simulink model "SiEngineCore"  (R2017b)
settings: Solver=VariableStepAuto  StartTime=0.0  StopTime=inf  RelTol=1e-3  EnableMultiTasking=on
model workspace (MAT data in the model file):
  AFRStoich = 14.6
  AirFilterArea = 0.000962112750162
  AirIntakeVol = 0.0137
  C_eng = 40000
  CompEff = [0.2 0.2 0.2 0.2 0.2 0.2 0.2 0.2 0.2 0.2 0.2 0.2 ... (5000 elements, 50x100)]
  CompMassFlwRate = [4.4091251837e-05 0.00441685548409 0.00879200250921 0.0131688186568 0.0175465480563 0.0219243905675 0.0263014996182 0.0306769799437 0.0350498852261 0.0394192156283 0.0437839152204 0.0481428692931 ... (5000 elements, 50x100)]
  CompPrsRatioBreakPoints = [1 1.02808080808 1.05616161616 1.08424242424 1.11232323232 1.1404040404 1.16848484848 1.19656565657 1.22464646465 1.25272727273 1.28080808081 1.30888888889 ... (100 elements, 1x100)]
  CompRefPrs = 101325
  CompRefTemp = 300
  CompSpdBreakPoints = [5 500.713942607 996.427885215 1492.14182782 1987.85577043 2483.56971304 2979.28365564 3474.99759825 3970.71154086 4466.42548347 4962.13942607 5457.85336868 ... (50 elements, 1x50)]
  CoolantTemp = 310
  Cps = 2
  ExhSysArea = 0.00138544236023
  ExhSysVol = 0.0044
  IcEffectiveness = 0.7
  InjSlp = 6.45161290323
  LHV = 47300000
  NCyl = 4
  Pstd = 101325
  Rair = 287
  Rexh = 297
  T_cool_start = 355
  T_coolnt_init = 355
  T_coolnt_max = 375
  ThrAngToC = [0  0.001; 90  0.735]
  ThrDiam = 50
  Tstd = 293.15
  TurbEff = [0.1 0.1 0.1 0.1 0.1 0.1 0.1 0.1 0.1 0.1 0.1 0.1 ... (3600 elements, 60x60)]
  TurbMassFlwRate = [0 0 0 0 0 0 0 0 0 0 0 0 ... (3600 elements, 60x60)]
  TurbPrsRatioBreakPoints = [1 1.0066198 1.0187236 1.0343974 1.0529583 1.0740113 1.0972904 1.1226 1.1497884 1.178734 1.2093357 1.2415084 ... (60 elements, 1x60)]
  TurbRefPres = 101325
  TurbRefTemp = 300
  TurbSpdBreakPoints = [0 236.716179913 473.432359826 710.148557878 946.864755929 1183.5809177 1420.29711576 1657.01327753 1893.72933048 2130.44574618 2367.16179913 2603.87821484 ... (60 elements, 60x1)]
  TurboInertia = 1.55e-05
  Vd = 0.0015
  Vexh = 0.0016
  Vint = 0.00286
  VolCompOut = 0.0026
  WgArea = 0.000314159265359
  cp_air = 1005
  cp_exh = 1005
  f_co = [6.86026635502e-05 6.86026635502e-05 0.000137130178455 0.000177313004818 0.000153545722458 0.000286109103754 0.00065603982686 0.00012726330728 0.000129286672759 0.000129286672759 0.000129286672759 0.000129286672759 ... (240 elements, 16x15)]
  f_co2 = [0.190124640361 0.190124640361 0.197310430134 0.198841052192 0.19976911847 0.200569885042 0.199664821109 0.20034918367 0.20035007673 0.20035007673 0.20035007673 0.20035007673 ... (240 elements, 16x15)]
  f_del_sa_bpt = [0 0.75 1.5 2.25 3 3.75 4.5 5.25 6 6.75 7.5 8.25 ... (65 elements, 1x65)]
  f_exhfrac_n_bpt = [750 1053.57142857 1357.14285714 1660.71428571 1964.28571429 2267.85714286 2571.42857143 2875 3178.57142857 3482.14285714 3785.71428571 4089.28571429 ... (15 elements, 1x15)]
  f_exhfrac_trq_bpt = [0 15 26.4285714286 37.8571428571 49.2857142857 60.7142857143 72.1428571429 83.5714285714 95 106.428571429 117.857142857 129.285714286 ... (16 elements, 1x16)]
  f_fric_temp_bpt = [274 276 278 280 282 284 286 288 290 292 294 296 ... (54 elements, 1x54)]
  f_fric_temp_mod = [3.96 3.22 2.56 2.26 2.11 2 1.9 1.83 1.76 1.7 1.65 1.6 ... (54 elements, 1x54)]
  f_hc = [0.00443209119576 0.00443209119576 0.00220684816441 0.00166684424867 0.00138421884093 0.0010658858934 0.00112857643245 0.00117703080332 0.00117597584116 0.00117597584116 0.00117597584116 0.00117597584116 ... (240 elements, 16x15)]
  f_m_lam = [0.94128 0.95565 0.97001 0.98437 0.99008 1.0004 0.97527 0.9549 0.92612 0.89735 0]
  f_m_lam_bpt = [0.65 0.7 0.75 0.8 0.85 0.9 0.95 1 1.05 1.1 2]
  f_m_sa = [1.0019 0.9988 0.9953 0.99173 0.98811 0.98441 0.98065 0.97682 0.97293 0.96897 0.96493 0.96083 ... (65 elements, 1x65)]
  f_mdot_air = [0 0 0 0 0 0 0 0 0 0 0 0 ... (400 elements, 20x20)]
  f_mdot_air_corr = [1.02156051768 1.00597426471 0.989411677851 1.0033499089 0.984591437857 0.988509040623 1.0326198627 1.02765527362 1.0134784519 0.998280021213 0.981755128787 0.967218261288 ... (400 elements, 20x20)]
  f_mdot_air_corr_ld_bpt = [0.223381333333 0.285105122807 0.346828912281 0.408552701754 0.470276491228 0.532000280702 0.593724070175 0.655447859649 0.717171649123 0.778895438596 0.84061922807 0.902343017544 ... (20 elements, 1x20)]
  f_mdot_air_ecp_bpt = [0 2.6316 5.2632 7.8947 10.5263 13.1579 15.7895 18.4211 21.0526 23.6842 26.3158 28.9474 ... (20 elements, 1x20)]
  f_mdot_air_n_bpt = [750 973.6842 1197.3684 1421.0526 1644.7368 1868.4211 2092.1053 2315.7895 2539.4737 2763.1579 2986.8421 3210.5263 ... (20 elements, 1x20)]
  f_mdot_trpd_bpt = [0 5.7895 11.5789 17.3684 23.1579 28.9474 34.7368 40.5263 46.3158 52.1053 57.8947 63.6842 ... (20 elements, 1x20)]
  f_nox = [4.08881357131e-05 4.08881357131e-05 0.00012346903723 0.000189339284589 0.00026637780763 0.000608287545555 0.00102018770254 0.00131576653087 0.00131610412986 0.00131610412986 0.00131610412986 0.00131610412986 ... (240 elements, 16x15)]
  f_nv = [0.64175366561 0.641419295169 0.640125365558 0.638690556197 0.644169906538 0.669178791311 0.731659452876 0.750078238889 0.750078238889 0.750078238889 0.750078238889 0.750078238889 ... (225 elements, 15x15)]
  f_nv_n_bpt = [750 1053.57142857 1357.14285714 1660.71428571 1964.28571429 2267.85714286 2571.42857143 2875 3178.57142857 3482.14285714 3785.71428571 4089.28571429 ... (15 elements, 1x15)]
  f_nv_prs_bpt = [31 40.6428571429 50.2857142857 59.9285714286 69.5714285714 79.2142857143 88.8571428571 98.5 108.142857143 117.785714286 127.428571429 137.071428571 ... (15 elements, 1x15)]
  f_sa_opt = [35.3085 35.3085 21.0105 10.3714 8.5076 7.1426 7.5656 -5.7766 -16.7061 -16.8345 -19.3546 -20.6085 ... (256 elements, 16x16)]
  f_t_exh = [739.936218766 750.584766028 772.770773797 791.235245621 803.106549716 885.862998064 920.498479307 920.498479307 920.498479307 920.498479307 920.498479307 920.498479307 ... (225 elements, 15x15)]
  f_t_exh_l_bpt = [0.2 0.275 0.35 0.425 0.5 0.575 0.65 0.725 0.8 0.875 0.95 1.025 ... (15 elements, 1x15)]
  f_t_exh_n_bpt = [750 1053.57142857 1357.14285714 1660.71428571 1964.28571429 2267.85714286 2571.42857143 2875 3178.57142857 3482.14285714 3785.71428571 4089.28571429 ... (15 elements, 1x15)]
  f_tm_corr = [0.839360054391 0.833393271885 0.82629554201 0.818442814437 0.811524387436 0.809164184856 0.814606352881 0.826887956871 0.842304598924 0.856886829014 0.869487025783 0.880530414174 ... (400 elements, 20x20)]
  f_tm_corr_n_bpt = [750 973.6842 1197.3684 1421.0526 1644.7368 1868.4211 2092.1053 2315.7895 2539.4737 2763.1579 2986.8421 3210.5263 ... (20 elements, 1x20)]
  f_tm_corr_nd_bpt = [0.3 0.38947 0.47895 0.56842 0.65789 0.74737 0.83684 0.92632 1.0158 1.1053 1.1947 1.2842 ... (20 elements, 1x20)]
  f_tq_fric = [0 0 0 0 0 0 0 0 0 0 0 0 ... (256 elements, 16x16)]
  f_tq_inr = [25.8508 25.8508 25.8508 25.8508 25.8508 25.8508 25.8508 25.8508 25.8508 25.8508 25.8508 25.8508 ... (256 elements, 16x16)]
  f_tq_inr_l_bpt = [0.1 0.2 0.28571 0.37143 0.45714 0.54286 0.62857 0.71429 0.8 0.88571 0.97143 1.0571 ... (16 elements, 1x16)]
  f_tq_inr_n_bpt = [0 750 1053.5714 1357.1429 1660.7143 1964.2857 2267.8571 2571.4286 2875 3178.5714 3482.1429 3785.7143 ... (16 elements, 1x16)]
  f_tq_nl = [15.0012133443 26.4298333923 37.8556656512 49.2846782956 60.7113978793 72.3451969202 77.459652163 78.5324534074 78.5324534074 78.5324534074 78.5324534074 78.5324534074 ... (225 elements, 15x15)]
  f_tq_nl_l_bpt = [0.2 0.275 0.35 0.425 0.5 0.575 0.65 0.725 0.8 0.875 0.95 1.025 ... (15 elements, 1x15)]
  f_tq_nl_n_bpt = [750 1053.57142857 1357.14285714 1660.71428571 1964.28571429 2267.85714286 2571.42857143 2875 3178.57142857 3482.14285714 3785.71428571 4089.28571429 ... (15 elements, 1x15)]
  f_tq_pump = [0 0 0 0 0 0 0 0 0 0 0 0 ... (256 elements, 16x16)]
  f_vivc = [0.37716 0.38164 0.38611 0.39033 0.39428 0.39795 0.40132 0.40441 0.40719 0.40967 0.41184 0.41372 ... (20 elements, 1x20)]
  f_vivc_icp_bpt = [0 2.6316 5.2632 7.8947 10.5263 13.1579 15.7895 18.4211 21.0526 23.6842 26.3158 28.9474 ... (20 elements, 1x20)]
  tau_cool = 3000
libraries: autolibfundflw x11, autolibboost x3, simulink x1, autolibcoreeng x1
(part 2 of 2)

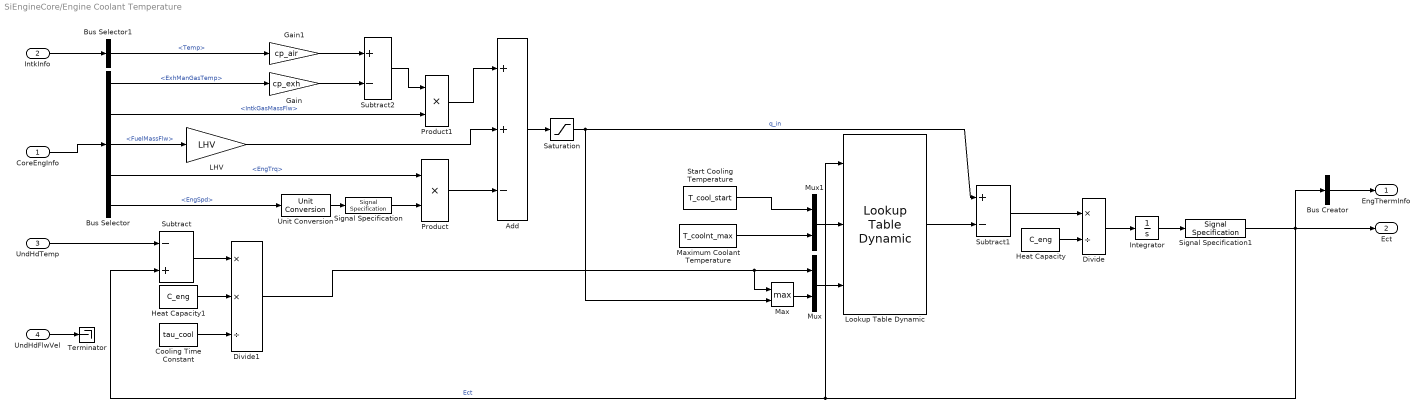
== system SiEngineCore/Engine Coolant Temperature ==
  CoreEngInfo : Inport
  IntkInfo : Inport  Port=2
  UndHdTemp : Inport  Port=3
  UndHdFlwVel : Inport  Port=4
  Add : Sum  Inputs=++-
  Bus Creator : BusCreator  Inputs=1
  Bus Selector : BusSelector  OutputSignals=ExhManGasTemp,IntkGasMassFlw,FuelMassFlw,EngTrq,EngSpd
  Bus Selector1 : BusSelector  OutputSignals=Vol.Temp
  Cooling Time Constant : Constant  Value=tau_cool
  Divide : Product  Inputs=*/
  Divide1 : Product  Inputs=**/
  Gain : Gain  Gain=cp_exh
  Gain1 : Gain  Gain=cp_air
  Heat Capacity : Constant  Value=C_eng
  Heat Capacity1 : Constant  Value=C_eng
  Integrator : Integrator  InitialCondition=T_coolnt_init  LimitOutput=on  UpperSaturationLimit=T_coolnt_max  LowerSaturationLimit=0  ZeroCross=off
  LHV : Gain  Gain=LHV
  Lookup Table Dynamic : simulink/Lookup Tables/Lookup Table Dynamic  LookUpMeth=Interpolation-Use End Values  OutDataType=fixdt('double')  OutScaling=[]  OutputDataTypeScalingMode=Specify via dialog  OutDataTypeStr=double  DoSatur=off
      settings: SourceProductName=Simulink
  Max : MinMax  Function=max  Inputs=2  ZeroCross=off
  Maximum Coolant Temperature : Constant  Value=T_coolnt_max
  Mux : Mux  Inputs=2
  Mux1 : Mux  Inputs=2
  Product : Product
  Product1 : Product
  Saturation : Saturate  UpperLimit=Inf  LowerLimit=0
  Signal Specification : SignalSpecification  Unit=rad/s
  Signal Specification1 : SignalSpecification  Unit=K
  Start Cooling Temperature : Constant  Value=T_cool_start
  Subtract : Sum  Inputs=-+
  Subtract1 : Sum  Inputs=+-
  Subtract2 : Sum  Inputs=+-
  Terminator : Terminator
  Unit Conversion : UnitConversion
  EngThermInfo : Outport  Unit=K
  Ect : Outport  Port=2  Unit=K
  wires:
  UndHdTemp/1 -> Subtract/1
  Heat Capacity/1 -> Divide/2
  Unit Conversion/1 -> Signal Specification/1
  Maximum Coolant Temperature/1 -> Mux1/2
  Signal Specification1/1 -> Subtract/2, Lookup Table Dynamic/1, Bus Creator/1, Ect/1  "Ect"
  UndHdFlwVel/1 -> Terminator/1
  Gain/1 -> Subtract2/2
  Bus Selector/4 -> Product/1  "<EngTrq>"
  Mux1/1 -> Lookup Table Dynamic/2
  Divide1/1 -> Max/1, Mux/1
  Heat Capacity1/1 -> Divide1/2
  Mux/1 -> Lookup Table Dynamic/3
  Start Cooling Temperature/1 -> Mux1/1
  Subtract/1 -> Divide1/1
  Saturation/1 -> Max/2, Subtract1/1  "q_in"
  Signal Specification/1 -> Product/2
  LHV/1 -> Add/2
  Product/1 -> Add/3
  Bus Selector/5 -> Unit Conversion/1  "<EngSpd>"
  Cooling Time Constant/1 -> Divide1/3
  CoreEngInfo/1 -> Bus Selector/1
  Bus Selector/3 -> LHV/1  "<FuelMassFlw>"
  Bus Selector/1 -> Gain/1  "<ExhManGasTemp>"
  Gain1/1 -> Subtract2/1
  Bus Selector1/1 -> Gain1/1  "<Temp>"
  Divide/1 -> Integrator/1
  Subtract1/1 -> Divide/1
  Lookup Table Dynamic/1 -> Subtract1/2
  Max/1 -> Mux/2
  Bus Creator/1 -> EngThermInfo/1
  IntkInfo/1 -> Bus Selector1/1
  Integrator/1 -> Signal Specification1/1
  Subtract2/1 -> Product1/1
  Bus Selector/2 -> Product1/2  "<IntkGasMassFlw>"
  Product1/1 -> Add/1
  Add/1 -> Saturation/1

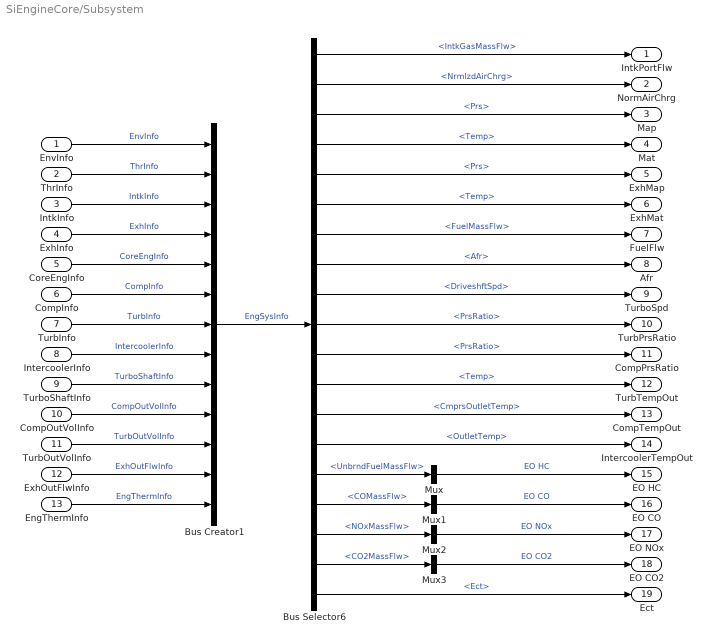
== system SiEngineCore/Subsystem ==
  EnvInfo : Inport
  ThrInfo : Inport  Port=2
  IntkInfo : Inport  Port=3
  ExhInfo : Inport  Port=4
  CoreEngInfo : Inport  Port=5
  CompInfo : Inport  Port=6
  TurbInfo : Inport  Port=7
  IntercoolerInfo : Inport  Port=8
  TurboShaftInfo : Inport  Port=9
  CompOutVolInfo : Inport  Port=10
  TurbOutVolInfo : Inport  Port=11
  ExhOutFlwInfo : Inport  Port=12
  EngThermInfo : Inport  Port=13
  Bus Creator1 : BusCreator  Inputs=13
  Bus Selector6 : BusSelector  OutputSignals=CoreEngInfo.IntkGasMassFlw,CoreEngInfo.NrmlzdAirChrg,IntkInfo.Vol.Prs,IntkInfo.Vol.Temp,ExhInfo.Vol.Prs,ExhInfo.Vol.Temp,CoreEngInfo.FuelMassFlw,CoreEngInfo.Afr,TurboShaftInfo.DriveshftSpd,TurbInfo.PrsRatio,CompInfo.PrsRatio,TurbOutVolInfo.Vol.Temp,CompInfo.CmprsOutletTemp,IntercoolerInfo.OutletTemp,ExhOutFlwInfo.Flw.Species.UnbrndFuelMassFlw,ExhOutFlwInfo.Flw.Species.COMassFlw,ExhOutFlwInfo.Flw.Species.NOxMassFlw,ExhOutFlwInfo.Flw.Species.CO2MassFlw,EngThermInfo.Ect
  Mux{,1..3} (4 alike) : Mux  Inputs=1
  IntkPortFlw : Outport
  NormAirChrg : Outport  Port=2  Unit=1
  Map : Outport  Port=3
  Mat : Outport  Port=4
  ExhMap : Outport  Port=5
  ExhMat : Outport  Port=6
  FuelFlw : Outport  Port=7
  Afr : Outport  Port=8  Unit=1
  TurboSpd : Outport  Port=9
  TurbPrsRatio : Outport  Port=10
  CompPrsRatio : Outport  Port=11
  TurbTempOut : Outport  Port=12
  CompTempOut : Outport  Port=13
  IntercoolerTempOut : Outport  Port=14
  EO HC : Outport  Port=15
  EO CO : Outport  Port=16
  EO NOx : Outport  Port=17
  EO CO2 : Outport  Port=18
  Ect : Outport  Port=19
  wires:
  CompInfo/1 -> Bus Creator1/6  "CompInfo"
  IntkInfo/1 -> Bus Creator1/3  "IntkInfo"
  ExhInfo/1 -> Bus Creator1/4  "ExhInfo"
  CoreEngInfo/1 -> Bus Creator1/5  "CoreEngInfo"
  EnvInfo/1 -> Bus Creator1/1  "EnvInfo"
  Bus Creator1/1 -> Bus Selector6/1  "EngSysInfo"
  ThrInfo/1 -> Bus Creator1/2  "ThrInfo"
  IntercoolerInfo/1 -> Bus Creator1/8  "IntercoolerInfo"
  TurbInfo/1 -> Bus Creator1/7  "TurbInfo"
  TurboShaftInfo/1 -> Bus Creator1/9  "TurboShaftInfo"
  Bus Selector6/1 -> IntkPortFlw/1  "<IntkGasMassFlw>"
  Bus Selector6/3 -> Map/1  "<Prs>"
  Bus Selector6/4 -> Mat/1  "<Temp>"
  Bus Selector6/5 -> ExhMap/1  "<Prs>"
  Bus Selector6/6 -> ExhMat/1  "<Temp>"
  Bus Selector6/7 -> FuelFlw/1  "<FuelMassFlw>"
  Bus Selector6/8 -> Afr/1  "<Afr>"
  Bus Selector6/2 -> NormAirChrg/1  "<NrmlzdAirChrg>"
  Bus Selector6/9 -> TurboSpd/1  "<DriveshftSpd>"
  Bus Selector6/10 -> TurbPrsRatio/1  "<PrsRatio>"
  Bus Selector6/11 -> CompPrsRatio/1  "<PrsRatio>"
  Bus Selector6/12 -> TurbTempOut/1  "<Temp>"
  Bus Selector6/13 -> CompTempOut/1  "<CmprsOutletTemp>"
  Bus Selector6/14 -> IntercoolerTempOut/1  "<OutletTemp>"
  CompOutVolInfo/1 -> Bus Creator1/10  "CompOutVolInfo"
  TurbOutVolInfo/1 -> Bus Creator1/11  "TurbOutVolInfo"
  ExhOutFlwInfo/1 -> Bus Creator1/12  "ExhOutFlwInfo"
  Mux/1 -> EO HC/1  "EO HC"
  Mux2/1 -> EO NOx/1  "EO NOx"
  Mux3/1 -> EO CO2/1  "EO CO2"
  Mux1/1 -> EO CO/1  "EO CO"
  Bus Selector6/15 -> Mux/1  "<UnbrndFuelMassFlw>"
  Bus Selector6/16 -> Mux1/1  "<COMassFlw>"
  Bus Selector6/17 -> Mux2/1  "<NOxMassFlw>"
  Bus Selector6/18 -> Mux3/1  "<CO2MassFlw>"
  Bus Selector6/19 -> Ect/1  "<Ect>"
  EngThermInfo/1 -> Bus Creator1/13  "EngThermInfo"
